simulink model "simulink_observateur"  (R2023a)
settings: Solver=VariableStepAuto  StartTime=0.0  StopTime=100  RelTol=1e-3
values from neighbouring files (symbols this model uses):
  A = [[0 0 1 0] ... (first row only)    [Code_main.m]
  B = transpose([0 0 1/M (-1)/(M*L)])    [Code_main.m]
  Cksi = [1 0 0 0]    [Code_main.m]
  K = lqr(A,B,Cksi'*Cksi,10)    [Code_main.m]
  L = (lqr(A',Cksi',B*B',1))'    [Code_main.m]
settings Model: Creator=bilheuxl  LastModifiedBy=bilheuxl

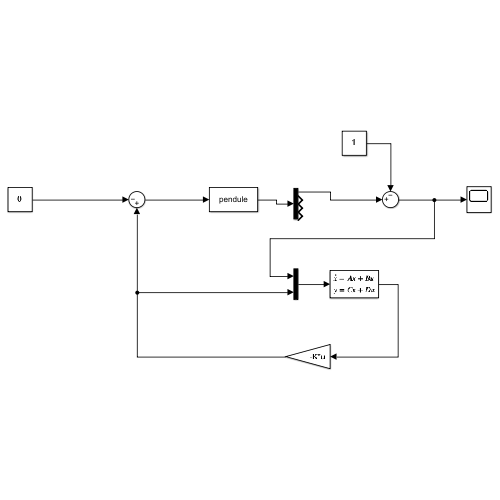
[thumbnail: Simulink's stored preview of the top-level diagram]
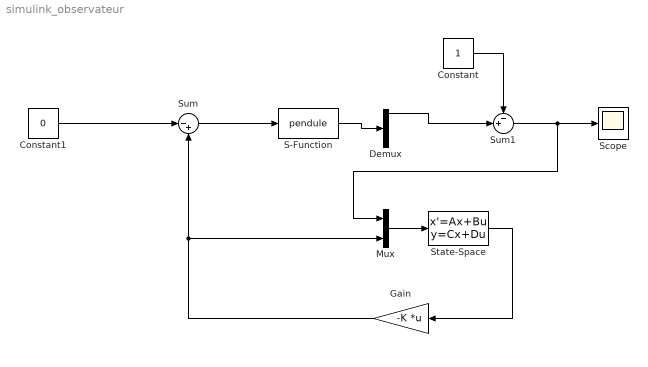
== system simulink_observateur ==
  Constant : Constant
  Constant1 : Constant  Value=0
  Demux : Demux
  Gain : Gain  Gain=-K  Multiplication=Matrix(K*u)
  Mux : Mux  Inputs=2
  S-Function : S-Function  FunctionName=pendule  SFunctionDeploymentMode=off  EnableBusSupport=off
  Scope : Scope
  State-Space : StateSpace  A=A-L*Cksi  B=[L B]  C=eye(4)  D=zeros(4, 2)  InitialCondition=transpose([2, 10*pi/180, 0, 0]) - transpose([1, 0, 0, 0])
  Sum : Sum  Inputs=|-+
  Sum1 : Sum  Inputs=-+|
  wires:
  Sum/1 -> S-Function/1
  Constant1/1 -> Sum/1
  Gain/1 -> Mux/2, Sum/2
  Sum1/1 -> Mux/1, Scope/1
  Constant/1 -> Sum1/1
  Mux/1 -> State-Space/1
  State-Space/1 -> Gain/1
  S-Function/1 -> Demux/1
  Demux/1 -> Sum1/2
